simulink model "SecRwLtStCalib"  (R2024b)
settings: Solver=FixedStepDiscrete  StartTime=0.0  StopTime=10.0  FixedStep=0.01  RelTol=1e-3
model workspace (MAT data in the model file):
  KeSMSwAcsMd6SecRwLtStBkReclnUpwdDnwdPos1Max_Val = Simulink.Parameter
  KeSMSwAcsMd6SecRwLtStBkReclnUpwdDnwdPos1Max_Val.Value = 1960
  KeSMSwAcsMd6SecRwLtStBkReclnUpwdDnwdPos1Max_Val.Complexity = 'real'
  KeSMSwAcsMd6SecRwLtStBkReclnUpwdDnwdPos1Max_Val.Dimensions = [1 1]
  KeSMSwAcsMd6SecRwLtStBkReclnUpwdDnwdPos1Max_Val.DataType = 'uint16'
  KeSMSwAcsMd6SecRwLtStBkReclnUpwdDnwdPos1Min_Val = Simulink.Parameter
  KeSMSwAcsMd6SecRwLtStBkReclnUpwdDnwdPos1Min_Val.Value = 1960
  KeSMSwAcsMd6SecRwLtStBkReclnUpwdDnwdPos1Min_Val.Complexity = 'real'
  KeSMSwAcsMd6SecRwLtStBkReclnUpwdDnwdPos1Min_Val.Dimensions = [1 1]
  KeSMSwAcsMd6SecRwLtStBkReclnUpwdDnwdPos1Min_Val.DataType = 'uint16'
  KeSMSwAcsMd6SecRwLtStBkReclnUpwdDnwdPos1_Val = Simulink.Parameter
  KeSMSwAcsMd6SecRwLtStBkReclnUpwdDnwdPos1_Val.Value = 1960
  KeSMSwAcsMd6SecRwLtStBkReclnUpwdDnwdPos1_Val.Complexity = 'real'
  KeSMSwAcsMd6SecRwLtStBkReclnUpwdDnwdPos1_Val.Dimensions = [1 1]
  KeSMSwAcsMd6SecRwLtStBkReclnUpwdDnwdPos1_Val.DataType = 'uint16'
  KeSMSwAcsMd6SecRwLtStBkReclnUpwdDnwdPosMax_Val = Simulink.Parameter
  KeSMSwAcsMd6SecRwLtStBkReclnUpwdDnwdPosMax_Val.Value = 1960
  KeSMSwAcsMd6SecRwLtStBkReclnUpwdDnwdPosMax_Val.Complexity = 'real'
  KeSMSwAcsMd6SecRwLtStBkReclnUpwdDnwdPosMax_Val.Dimensions = [1 1]
  KeSMSwAcsMd6SecRwLtStBkReclnUpwdDnwdPosMax_Val.DataType = 'uint16'
  KeSMSwAcsMd6SecRwLtStBkReclnUpwdDnwdPosMin_Val = Simulink.Parameter
  KeSMSwAcsMd6SecRwLtStBkReclnUpwdDnwdPosMin_Val.Value = 1960
  KeSMSwAcsMd6SecRwLtStBkReclnUpwdDnwdPosMin_Val.Complexity = 'real'
  KeSMSwAcsMd6SecRwLtStBkReclnUpwdDnwdPosMin_Val.Dimensions = [1 1]
  KeSMSwAcsMd6SecRwLtStBkReclnUpwdDnwdPosMin_Val.DataType = 'uint16'
  KeSMSwAcsMd6SecRwLtStBkReclnUpwdDnwdPos_Val = Simulink.Parameter
  KeSMSwAcsMd6SecRwLtStBkReclnUpwdDnwdPos_Val.Value = 1960
  KeSMSwAcsMd6SecRwLtStBkReclnUpwdDnwdPos_Val.Complexity = 'real'
  KeSMSwAcsMd6SecRwLtStBkReclnUpwdDnwdPos_Val.Dimensions = [1 1]
  KeSMSwAcsMd6SecRwLtStBkReclnUpwdDnwdPos_Val.DataType = 'uint16'
undefined symbols (not defined in the file or in its folder): KeSMSw4SAcsMd21SecRwLtStBkReclnUpwdDnwdPos_Val, KeSMSw4SAcsMd21SecRwLtStBkReclnUpwdDnwdPosMax_Val, KeSMSw4SAcsMd21SecRwLtStBkReclnUpwdDnwdPosMin_Val, KeSMSw4SAcsMd21SecRwLtStFrwdBkwdPos_Val, KeSMSw4SAcsMd21SecRwLtStFrwdBkwdPosMax_Val, KeSMSw4SAcsMd21SecRwLtStFrwdBkwdPosMin_Val, KeSMSw4SAcsMd21SecRwLtStHdrstFrwdBkwdPos_Val, KeSMSw4SAcsMd21SecRwLtStHdrstFrwdBkwdPosMax_Val, KeSMSw4SAcsMd21SecRwLtStHdrstFrwdBkwdPosMin_Val, KeSMSw4SAcsMd21SecRwLtStHdrstUpwdDnwdPos_Val, KeSMSw4SAcsMd21SecRwLtStHdrstUpwdDnwdPosMax_Val, KeSMSw4SAcsMd21SecRwLtStHdrstUpwdDnwdPosMin_Val, KeSMSw4SAcsMd22SecRwLtStBkReclnUpwdDnwdPos1_Val, KeSMSw4SAcsMd22SecRwLtStBkReclnUpwdDnwdPos2_Val, KeSMSw4SAcsMd22SecRwLtStBkReclnUpwdDnwdPos2Max_Val, KeSMSw4SAcsMd22SecRwLtStBkReclnUpwdDnwdPos2Min_Val, KeSMSw4SAcsMd22SecRwLtStBkReclnUpwdDnwdPosMax_Val, KeSMSw4SAcsMd22SecRwLtStBkReclnUpwdDnwdPosMin_Val, KeSMSw4SAcsMd22SecRwLtStFrwdBkwdPos_Val, KeSMSw4SAcsMd22SecRwLtStFrwdBkwdPosMax_Val, KeSMSw4SAcsMd22SecRwLtStFrwdBkwdPosMin_Val, KeSMSw4SAcsMd22SecRwLtStFtrstUpwdDnwdPos_Val, KeSMSw4SAcsMd22SecRwLtStFtrstUpwdDnwdPosMax_Val, KeSMSw4SAcsMd22SecRwLtStFtrstUpwdDnwdPosMin_Val, KeSMSw4SAcsMd22SecRwLtStHdrstFrwdBkwdPos_Val, KeSMSw4SAcsMd22SecRwLtStHdrstFrwdBkwdPosMax_Val, KeSMSw4SAcsMd22SecRwLtStHdrstFrwdBkwdPosMin_Val, KeSMSw4SAcsMd22SecRwLtStHdrstUpwdDnwdPos_Val, KeSMSw4SAcsMd22SecRwLtStHdrstUpwdDnwdPosMax_Val, KeSMSw4SAcsMd22SecRwLtStHdrstUpwdDnwdPosMin_Val, KeSMSw4SAcsMd22SecRwLtStLegrstOtwdInwdPos_Val, KeSMSw4SAcsMd22SecRwLtStLegrstOtwdInwdPosMax_Val, KeSMSw4SAcsMd22SecRwLtStLegrstOtwdInwdPosMin_Val, KeSMSw4SAcsMd22SecRwLtStLegrstUpwdDnwdPos_Val, KeSMSw4SAcsMd22SecRwLtStLegrstUpwdDnwdPosMax_Val, KeSMSw4SAcsMd22SecRwLtStLegrstUpwdDnwdPosMin_Val, KeSMSw4SAcsMd25SecRwLtStBkReclnUpwdDnwdPos_Val, KeSMSw4SAcsMd25SecRwLtStBkReclnUpwdDnwdPosMax_Val, KeSMSw4SAcsMd25SecRwLtStBkReclnUpwdDnwdPosMin_Val, KeSMSw4SAcsMd25SecRwLtStFrwdBkwdPos_Val, KeSMSw4SAcsMd25SecRwLtStFrwdBkwdPosMax_Val, KeSMSw4SAcsMd25SecRwLtStFrwdBkwdPosMin_Val, KeSMSw4SAcsMd25SecRwLtStHdrstFrwdBkwdPos_Val, KeSMSw4SAcsMd25SecRwLtStHdrstFrwdBkwdPosMax_Val, KeSMSw4SAcsMd25SecRwLtStHdrstFrwdBkwdPosMin_Val, KeSMSw4SAcsMd25SecRwLtStHdrstUpwdDnwdPos_Val, KeSMSw4SAcsMd25SecRwLtStHdrstUpwdDnwdPosMax_Val, KeSMSw4SAcsMd25SecRwLtStHdrstUpwdDnwdPosMin_Val, KeSMSw4SAcsMd26SecRwLtStBkReclnUpwdDnwdPos_Val, KeSMSw4SAcsMd26SecRwLtStBkReclnUpwdDnwdPosMax_Val, KeSMSw4SAcsMd26SecRwLtStBkReclnUpwdDnwdPosMin_Val, KeSMSw4SAcsMd26SecRwLtStFrwdBkwdPos_Val, KeSMSw4SAcsMd26SecRwLtStFrwdBkwdPosMax_Val, KeSMSw4SAcsMd26SecRwLtStFrwdBkwdPosMin_Val, KeSMSw4SAcsMd26SecRwLtStFtrstUpwdDnwdPos_Val, KeSMSw4SAcsMd26SecRwLtStFtrstUpwdDnwdPosMax_Val, KeSMSw4SAcsMd26SecRwLtStFtrstUpwdDnwdPosMin_Val, KeSMSw4SAcsMd26SecRwLtStHdrstFrwdBkwdPos_Val, KeSMSw4SAcsMd26SecRwLtStHdrstFrwdBkwdPosMax_Val, KeSMSw4SAcsMd26SecRwLtStHdrstFrwdBkwdPosMin_Val ... (+496)
libraries: TrgtPosSelcLib x61, StIsPosChkLib x1, simulink x1
(part 1 of 8)
settings Model: ParameterArgumentNames=KeSMSwAcsMd6SecRwLtStBkReclnUpwdDnwdPos1Max_Val,KeSMSwAcsMd6SecRwLtStBkReclnUpwdDnwdPos1Min_Val,KeSMSwAcsMd6SecRwLtStBkReclnUpwdDnwdPos1_Val,KeSMSwAcsMd6SecRwLtStBkReclnUpwdDnwdPosMax_Val,KeSMSwAcsMd6SecRwLtStBkReclnUpwdDnwdPosMin_Val,KeSMSwAcsMd6SecRwLtStBkReclnUpwdDnwdPos_Val  Creator=sn2xws  LastModifiedBy=sn55gm
settings Model: ModifiedHistory=|
  | 2024.10.15 V3.0.0 新增Bitmask接口
  | 2024.10.29 V3.0.1 6s版本Md1 Md56靠背不应选择Cal1
  | 2024.12.12 V3.0.2 增加三排靠背折叠的判断余量
  | 25.7.1 V3.13.0 增加Md61 Md62
settings SolverCC: AlgebraicLoopSolver=TrustRegion
settings DataIOCC: SaveFormat=StructureWithTime  ReturnWorkspaceOutputs=off
settings OptimizationCC: DefaultParameterBehavior=Inlined  EnhancedBackFolding=on  PassReuseOutputArgsAs=Individual arguments  ZeroExternalMemoryAtStartup=off  ZeroInternalMemoryAtStartup=off  OptimizeBlockOrder=speed  DifferentSizesBufferReuse=on  OptimizationCustomize=off  EfficientTunableParamExpr=on
settings DebuggingCC: ParameterTunabilityLossMsg=error  UnconnectedInputMsg=warning  UnconnectedOutputMsg=warning  UnconnectedLineMsg=warning  ArithmeticOperatorsInVariantConditions=warning
settings ModelReferenceCC: EnableRefExpFcnMdlSchedulingChecks=on  ModelReferenceNumInstancesAllowed=Single
settings SFSimCC: MATLABDynamicMemAlloc=off  CustomCodeUndefinedFunction=UseInterfaceOnly
settings RTWCC: Description=AUTOSAR  SystemTargetFile=autosar.tlc  GenCodeOnly=on  TemplateMakefile=ert_default_tmf  GenerateReport=on  IncludeHyperlinkInReport=on  LaunchReport=on  DataTypeReplacement=CDataTypesFixedWidth  GenerateTraceInfo=on  GenerateTraceReport=on  GenerateTraceReportSl=on  GenerateTraceReportSf=on  GenerateTraceReportEml=on  GPUComputeCapability=3.5
settings CodeAppCC: ForceParamTrailComments=on  IgnoreCustomStorageClasses=off  OperatorAnnotations=on  SimulinkDataObjDesc=on  SFDataObjDesc=on  InsertBlockDesc=on
settings STFCustomTargetCC: TargetLangStandard=C99 (ISO)  MultiwordLength=256  ParMdlRefBuildCompliant=on  CompOptLevelCompliant=on  IncludeMdlTerminateFcn=off  CombineOutputUpdateFcns=on  SuppressErrorStatus=on  ERTCustomFileBanners=on  SupportNonFinite=off  SupportComplex=off  SupportContinuousTime=off  SupportNonInlinedSFcns=off  RemoveResetFunc=on  MATLABClassNameForMDSCustomization=Simulink.SoftwareTarget.ERTCustomization  AutosarCompliant=on  UseToolchainInfoCompliant=on  LookupTableObjectStructAxisOrder=2,1,3,4,...  LUTObjectStructOrderEvenSpacing=Size,Table,Breakpoints  SystemTargetFile=autosar.tlc
settings ERTTargetCC: TargetLangStandard=C99 (ISO)  ConcurrentExecutionCompliant=off  IncludeMdlTerminateFcn=off  SuppressErrorStatus=on  SupportNonFinite=off  SupportComplex=off  ModelStepFunctionPrototypeControlCompliant=off  CPPClassGenCompliant=off  AutosarCompliant=on  LookupTableObjectStructAxisOrder=2,1,3,4,...  LUTObjectStructOrderEvenSpacing=Size,Table,Breakpoints  ERTCustomFileTemplate=example_file_process.tlc  ERTFilePackagingFormat=Compact  BooleanTrueId=TRUE  BooleanFalseId=FALSE  DynamicArrayContainerType=coder::array

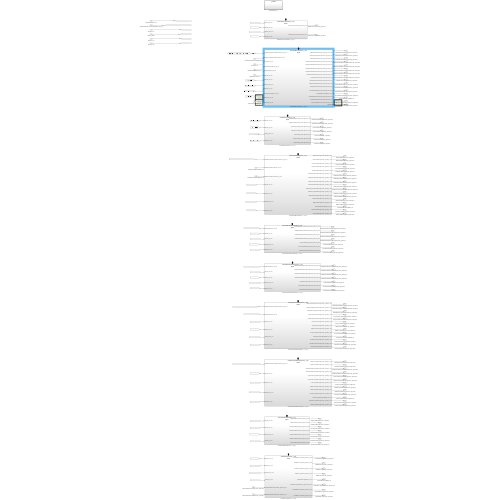
[thumbnail: Simulink's stored preview of the top-level diagram]
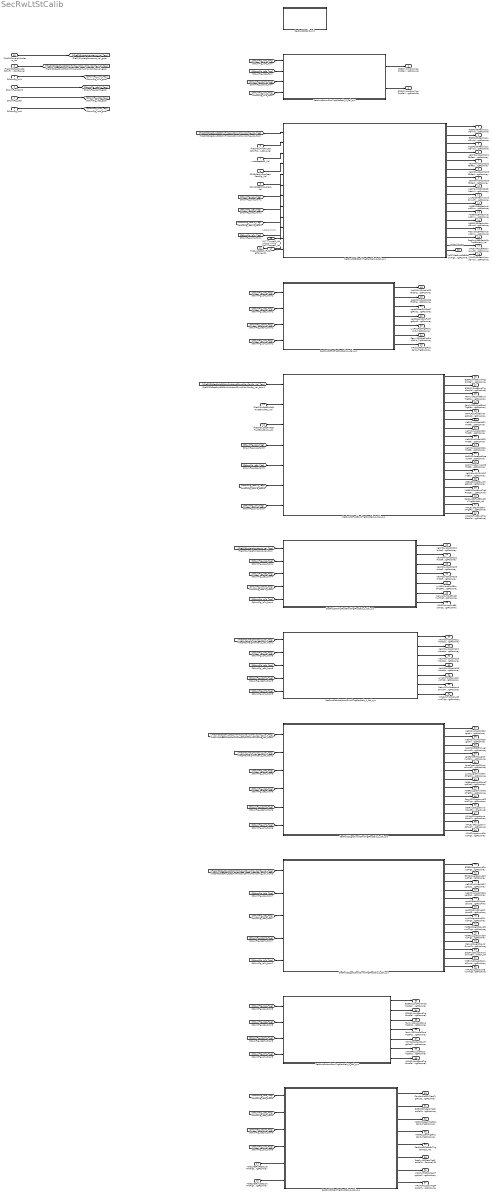
== system SecRwLtStCalib ==
  note: Added blocks
  note: Added blocks
  note: Added blocks
  StNumFlg_Is4s : Inport  OutDataTypeStr=boolean  PortDimensions=1
  StNumFlg_Is6s : Inport  Port=2  OutDataTypeStr=boolean  PortDimensions=1
  StNumFlg_Is6s7s : Inport  Port=3  OutDataTypeStr=boolean  PortDimensions=1
  StNumFlg_Is7s : Inport  Port=4  OutDataTypeStr=boolean  PortDimensions=1
  IfVeSMSbSecRwLtStCshnFrntUpwdDnwdMovConfig_Val : Inport  Port=5  OutDataTypeStr=boolean  PortDimensions=1
  IfVeSMSuThdRwLtStCshnFldUpwdDnwdPos_Val : Inport  Port=6  OutDataTypeStr=uint16  PortDimensions=1
  modestate32_Val : Inport  Port=7  OutDataTypeStr=uint32  PortDimensions=1
  R2LBkReclinFirstStepPassFlg_Val : Inport  Port=8  OutDataTypeStr=boolean  PortDimensions=1
  R2LMdSeatOccupied_Val : Inport  Port=9  OutDataTypeStr=boolean  PortDimensions=1
  ThdRwLtStCshnFldStgDone_Val : Inport  Port=10  OutDataTypeStr=boolean  PortDimensions=1
  IfVeSMSuSecRwRtStFrwdBkwdPos_Val : Inport  Port=11  OutDataTypeStr=uint16  PortDimensions=1
  IfVeSMSuSecRwRtStFrwdBkwdPosV_Val : Inport  Port=12  OutDataTypeStr=boolean  PortDimensions=1
  IfVeSMSuHeightIndexLt_Val : Inport  Description=|  Port=13  OutDataTypeStr=uint8  PortDimensions=1
      | 0：under 160
      | 1：160
      | 2：165
      | 3：170
      | 4：175
      | 5：180
      | 6：over 180
  Md61SecRwRtStCushFrntTrgtPosCalib_TrgtPosArray : Inport  Description=|  Port=14  OutDataTypeStr=uint16  PortDimensions=3
      | 0:Pos
      | 1:Max
      | 2:Min
  Md62SecRwLtStCushFrntTrgtPosCalib_TrgtPosArray : Inport  Description=|  Port=15  OutDataTypeStr=uint16  PortDimensions=3
      | 0:Pos
      | 1:Max
      | 2:Min
  Md27Target1_Val : Inport  Port=16  OutDataTypeStr=boolean  PortDimensions=1
  Md27Target2_Val : Inport  Port=17  OutDataTypeStr=boolean  PortDimensions=1
  SecRwLtStArmScrnTrgtPosSelc_1_Cal_sys : Subsystem
  SecRwLtStBkReclnTrgtPosSelc_1_Cal_sys : Subsystem
  SecRwLtStCalib_Init : Subsystem
  SecRwLtStFtrstTrgtPosSelc_1_Cal_sys : Subsystem
  SecRwLtStFwdBkwdTrgtPosSelc_1_Cal_sys : Subsystem
  SecRwLtStHdrstFwdBkwdTrgtPosSelc_1_Cal_sys : Subsystem
  SecRwLtStHdrstUpwdDnwdTrgtPosSelc_1_Cal_sys : Subsystem
  SecRwLtStLgrstInwdOtwdTrgtPosSelc_1_Cal_sys : Subsystem
  SecRwLtStLgrstUpwdDnwdTrgtPosSelc_1_Cal_sys : Subsystem
  SecRwLtStLtwdRtwdTrgtPosSelc_1_Cal_sys : Subsystem
  SecRwLtStZeroTrgtPosSelc_1_Cal_sys : Subsystem
  EZER2LArmScrnTrgtPosCalib_TrgtPosArray : Outport  Description=|  OutDataTypeStr=uint16  PortDimensions=3  VectorParamsAs1DForOutWhenUnconnected=off
      | 0:Pos
      | 1:Max
      | 2:Min
  EZQR2LArmScrnTrgtPosCalib_TrgtPosArray : Outport  Description=|  Port=2  OutDataTypeStr=uint16  PortDimensions=3  VectorParamsAs1DForOutWhenUnconnected=off
      | 0:Pos
      | 1:Max
      | 2:Min
  EZER2LBkReclnUpwdDnwdTrgtPosCalib_TrgtPosArray : Outport  Description=|  Port=3  OutDataTypeStr=uint16  PortDimensions=3  VectorParamsAs1DForOutWhenUnconnected=off
      | 0:Pos
      | 1:Max
      | 2:Min
  EZER2LBkReclnUpwdDnwdTrgtPosCalib1_TrgtPosArray : Outport  Description=|  Port=4  OutDataTypeStr=uint16  PortDimensions=3  VectorParamsAs1DForOutWhenUnconnected=off
      | 0:Pos
      | 1:Max
      | 2:Min
  EZQR2LBkReclnUpwdDnwdTrgtPosCalib_TrgtPosArray : Outport  Description=|  Port=5  OutDataTypeStr=uint16  PortDimensions=3  VectorParamsAs1DForOutWhenUnconnected=off
      | 0:Pos
      | 1:Max
      | 2:Min
  KeSMSw4SAcsMd21BkReclnUpwdDnwdTrgtPosCalib_TrgtPosArray : Outport  Description=|  Port=6  OutDataTypeStr=uint16  PortDimensions=3  VectorParamsAs1DForOutWhenUnconnected=off
      | 0:Pos
      | 1:Max
      | 2:Min
  KeSMSw4SAcsMd22BkReclnUpwdDnwdTrgtPosCalib_TrgtPosArray : Outport  Description=|  Port=7  OutDataTypeStr=uint16  PortDimensions=3  VectorParamsAs1DForOutWhenUnconnected=off
      | 0:Pos
      | 1:Max
      | 2:Min
  KeSMSw4SAcsMd25BkReclnUpwdDnwdTrgtPosCalib_TrgtPosArray : Outport  Description=|  Port=8  OutDataTypeStr=uint16  PortDimensions=3  VectorParamsAs1DForOutWhenUnconnected=off
      | 0:Pos
      | 1:Max
      | 2:Min
  KeSMSw4SAcsMd26BkReclnUpwdDnwdTrgtPosCalib_TrgtPosArray : Outport  Description=|  Port=9  OutDataTypeStr=uint16  PortDimensions=3  VectorParamsAs1DForOutWhenUnconnected=off
      | 0:Pos
      | 1:Max
      | 2:Min
  KeSMSwMd32R2LBkReclnUpwdDnwdTrgtPosCalib_TrgtPosArray : Outport  Description=|  Port=10  OutDataTypeStr=uint16  PortDimensions=3  VectorParamsAs1DForOutWhenUnconnected=off
      | 0:Pos
      | 1:Max
      | 2:Min
  LyLR2LBkReclnUpwdDnwdTrgtPosCalib_TrgtPosArray : Outport  Description=|  Port=11  OutDataTypeStr=uint16  PortDimensions=3  VectorParamsAs1DForOutWhenUnconnected=off
      | 0:Pos
      | 1:Max
      | 2:Min
  Md56R2LBkReclnUpwdDnwdTrgtPosCalib_TrgtPosArray : Outport  Description=|  Port=12  OutDataTypeStr=uint16  PortDimensions=3  VectorParamsAs1DForOutWhenUnconnected=off
      | 0:Pos
      | 1:Max
      | 2:Min
  Md56R2LBkReclnUpwdDnwdTrgtPosCalib1_TrgtPosArray : Outport  Description=|  Port=13  OutDataTypeStr=uint16  PortDimensions=3  VectorParamsAs1DForOutWhenUnconnected=off
      | 0:Pos
      | 1:Max
      | 2:Min
  Md8R2LBkReclnUpwdDnwdTrgtPosCalib_TrgtPosArray : Outport  Description=|  Port=14  OutDataTypeStr=uint16  PortDimensions=3  VectorParamsAs1DForOutWhenUnconnected=off
      | 0:Pos
      | 1:Max
      | 2:Min
  RecvLR2LBkReclnUpwdDnwdTrgtPosCalib_TrgtPosArray : Outport  Description=|  Port=15  OutDataTypeStr=uint16  PortDimensions=3  VectorParamsAs1DForOutWhenUnconnected=off
      | 0:Pos
      | 1:Max
      | 2:Min
  SecRwLtStBkReclnEnTrigBitMask_Val : Outport  Port=16  OutDataTypeStr=uint32  PortDimensions=1  VectorParamsAs1DForOutWhenUnconnected=off
  VIPLExitR2LBkReclnUpwdDnwdTrgtPosCalib_TrgtPosArray : Outport  Description=|  Port=17  OutDataTypeStr=uint16  PortDimensions=3  VectorParamsAs1DForOutWhenUnconnected=off
      | 0:Pos
      | 1:Max
      | 2:Min
  VIPLR2LBkReclnUpwdDnwdTrgtPosCalib_TrgtPosArray : Outport  Description=|  Port=18  OutDataTypeStr=uint16  PortDimensions=3  VectorParamsAs1DForOutWhenUnconnected=off
      | 0:Pos
      | 1:Max
      | 2:Min
  KeSMSw4SAcsMd22FtrstTrgtPosCalib_TrgtPosArray : Outport  Description=|  Port=19  OutDataTypeStr=uint16  PortDimensions=3  VectorParamsAs1DForOutWhenUnconnected=off
      | 0:Pos
      | 1:Max
      | 2:Min
  KeSMSw4SAcsMd26FtrstTrgtPosCalib_TrgtPosArray : Outport  Description=|  Port=20  OutDataTypeStr=uint16  PortDimensions=3  VectorParamsAs1DForOutWhenUnconnected=off
      | 0:Pos
      | 1:Max
      | 2:Min
  LgrstCloseLR2LFtrstTrgtPosCalib_TrgtPosArray : Outport  Description=|  Port=21  OutDataTypeStr=uint16  PortDimensions=3  VectorParamsAs1DForOutWhenUnconnected=off
      | 0:Pos
      | 1:Max
      | 2:Min
  LgrstOpenLR2LFtrstTrgtPosCalib_TrgtPosArray : Outport  Description=|  Port=22  OutDataTypeStr=uint16  PortDimensions=3  VectorParamsAs1DForOutWhenUnconnected=off
      | 0:Pos
      | 1:Max
      | 2:Min
  LyLR2LFtrstTrgtPosCalib_TrgtPosArray : Outport  Description=|  Port=23  OutDataTypeStr=uint16  PortDimensions=3  VectorParamsAs1DForOutWhenUnconnected=off
      | 0:Pos
      | 1:Max
      | 2:Min
  RecvLR2LFtrstTrgtPosCalib_TrgtPosArray : Outport  Description=|  Port=24  OutDataTypeStr=uint16  PortDimensions=3  VectorParamsAs1DForOutWhenUnconnected=off
      | 0:Pos
      | 1:Max
      | 2:Min
  VIPLR2LFtrstTrgtPosCalib_TrgtPosArray : Outport  Description=|  Port=25  OutDataTypeStr=uint16  PortDimensions=3  VectorParamsAs1DForOutWhenUnconnected=off
      | 0:Pos
      | 1:Max
      | 2:Min
  EZER2LFwdBkwdTrgtPosCalib_TrgtPosArray : Outport  Description=|  Port=26  OutDataTypeStr=uint16  PortDimensions=3  VectorParamsAs1DForOutWhenUnconnected=off
      | 0:Pos
      | 1:Max
      | 2:Min
  EZQR2LFwdBkwdTrgtPosCalib_TrgtPosArray : Outport  Description=|  Port=27  OutDataTypeStr=uint16  PortDimensions=3  VectorParamsAs1DForOutWhenUnconnected=off
      | 0:Pos
      | 1:Max
      | 2:Min
  FamlyLR2LFwdBkwdTrgtPosCalib_TrgtPosArray : Outport  Description=|  Port=28  OutDataTypeStr=uint16  PortDimensions=3  VectorParamsAs1DForOutWhenUnconnected=off
      | 0:Pos
      | 1:Max
      | 2:Min
  FamlyRR2LFwdBkwdTrgtPosCalib_TrgtPosArray : Outport  Description=|  Port=29  OutDataTypeStr=uint16  PortDimensions=3  VectorParamsAs1DForOutWhenUnconnected=off
      | 0:Pos
      | 1:Max
      | 2:Min
  INTMLR2LFwdBkwdTrgtPosCalib_TrgtPosArray : Outport  Description=|  Port=30  OutDataTypeStr=uint16  PortDimensions=3  VectorParamsAs1DForOutWhenUnconnected=off
      | 0:Pos
      | 1:Max
      | 2:Min
  KeSMSw4SAcsMd21FwdBkwdTrgtPosCalib_TrgtPosArray : Outport  Description=|  Port=31  OutDataTypeStr=uint16  PortDimensions=3  VectorParamsAs1DForOutWhenUnconnected=off
      | 0:Pos
      | 1:Max
      | 2:Min
  KeSMSw4SAcsMd22FwdBkwdTrgtPosCalib_TrgtPosArray : Outport  Description=|  Port=32  OutDataTypeStr=uint16  PortDimensions=3  VectorParamsAs1DForOutWhenUnconnected=off
      | 0:Pos
      | 1:Max
      | 2:Min
  KeSMSw4SAcsMd25FwdBkwdTrgtPosCalib_TrgtPosArray : Outport  Description=|  Port=33  OutDataTypeStr=uint16  PortDimensions=3  VectorParamsAs1DForOutWhenUnconnected=off
      | 0:Pos
      | 1:Max
      | 2:Min
  KeSMSw4SAcsMd26FwdBkwdTrgtPosCalib_TrgtPosArray : Outport  Description=|  Port=34  OutDataTypeStr=uint16  PortDimensions=3  VectorParamsAs1DForOutWhenUnconnected=off
      | 0:Pos
      | 1:Max
      | 2:Min
  KeSMSw4sLegrstOpenLMdFwdBkwdTrgtPosCalib_TrgtPosArray : Outport  Description=|  Port=35  OutDataTypeStr=uint16  PortDimensions=3  VectorParamsAs1DForOutWhenUnconnected=off
      | 0:Pos
      | 1:Max
      | 2:Min
  KeSMSw4SLyingLMDFwdBkwdTrgtPosCalib_TrgtPosArray : Outport  Description=|  Port=36  OutDataTypeStr=uint16  PortDimensions=3  VectorParamsAs1DForOutWhenUnconnected=off
      | 0:Pos
      | 1:Max
      | 2:Min
  KeSMSw4SVIPLMDFwdBkwdTrgtPosCalib_TrgtPosArray : Outport  Description=|  Port=37  OutDataTypeStr=uint16  PortDimensions=3  VectorParamsAs1DForOutWhenUnconnected=off
      | 0:Pos
      | 1:Max
      | 2:Min
  Md56R2LFwdBkwdTrgtPosCalib_TrgtPosArray : Outport  Description=|  Port=38  OutDataTypeStr=uint16  PortDimensions=3  VectorParamsAs1DForOutWhenUnconnected=off
      | 0:Pos
      | 1:Max
      | 2:Min
  Md8R2LFwdBkwdTrgtPosCalib_TrgtPosArray : Outport  Description=|  Port=39  OutDataTypeStr=uint16  PortDimensions=3  VectorParamsAs1DForOutWhenUnconnected=off
      | 0:Pos
      | 1:Max
      | 2:Min
  SecRwLtStFwdBkwdEnTrigBitMask_Val : Outport  Port=40  OutDataTypeStr=uint32  PortDimensions=1  VectorParamsAs1DForOutWhenUnconnected=off
  VIPLExitR2LFwdBkwdTrgtPosCalib_TrgtPosArray : Outport  Description=|  Port=41  OutDataTypeStr=uint16  PortDimensions=3  VectorParamsAs1DForOutWhenUnconnected=off
      | 0:Pos
      | 1:Max
      | 2:Min
  VIPLR2LFwdBkwdTrgtPosCalib_TrgtPosArray : Outport  Description=|  Port=42  OutDataTypeStr=uint16  PortDimensions=3  VectorParamsAs1DForOutWhenUnconnected=off
      | 0:Pos
      | 1:Max
      | 2:Min
  KeSMSw4SAcsMd21HdrstFwdBkwdTrgtPosCalib_TrgtPosArray : Outport  Description=|  Port=43  OutDataTypeStr=uint16  PortDimensions=3  VectorParamsAs1DForOutWhenUnconnected=off
      | 0:Pos
      | 1:Max
      | 2:Min
  KeSMSw4SAcsMd22HdrstFwdBkwdTrgtPosCalib_TrgtPosArray : Outport  Description=|  Port=44  OutDataTypeStr=uint16  PortDimensions=3  VectorParamsAs1DForOutWhenUnconnected=off
      | 0:Pos
      | 1:Max
      | 2:Min
  KeSMSw4SAcsMd25HdrstFwdBkwdTrgtPosCalib_TrgtPosArray : Outport  Description=|  Port=45  OutDataTypeStr=uint16  PortDimensions=3  VectorParamsAs1DForOutWhenUnconnected=off
      | 0:Pos
      | 1:Max
      | 2:Min
  KeSMSw4SAcsMd26HdrstFwdBkwdTrgtPosCalib_TrgtPosArray : Outport  Description=|  Port=46  OutDataTypeStr=uint16  PortDimensions=3  VectorParamsAs1DForOutWhenUnconnected=off
      | 0:Pos
      | 1:Max
      | 2:Min
  LyLR2LHdrstFwdBkwdTrgtPosCalib_TrgtPosArray : Outport  Description=|  Port=47  OutDataTypeStr=uint16  PortDimensions=3  VectorParamsAs1DForOutWhenUnconnected=off
      | 0:Pos
      | 1:Max
      | 2:Min
  RecvLR2LHdrstFwdBkwdTrgtPosCalib_TrgtPosArray : Outport  Description=|  Port=48  OutDataTypeStr=uint16  PortDimensions=3  VectorParamsAs1DForOutWhenUnconnected=off
      | 0:Pos
      | 1:Max
      | 2:Min
  VIPLR2LHdrstFwdBkwdTrgtPosCalib_TrgtPosArray : Outport  Description=|  Port=49  OutDataTypeStr=uint16  PortDimensions=3  VectorParamsAs1DForOutWhenUnconnected=off
      | 0:Pos
      | 1:Max
      | 2:Min
  KeSMSw4SAcsMd21HdrstUpwdDnwdTrgtPosCalib_TrgtPosArray : Outport  Description=|  Port=50  OutDataTypeStr=uint16  PortDimensions=3  VectorParamsAs1DForOutWhenUnconnected=off
      | 0:Pos
      | 1:Max
      | 2:Min
  KeSMSw4SAcsMd22HdrstUpwdDnwdTrgtPosCalib_TrgtPosArray : Outport  Description=|  Port=51  OutDataTypeStr=uint16  PortDimensions=3  VectorParamsAs1DForOutWhenUnconnected=off
      | 0:Pos
      | 1:Max
      | 2:Min
  KeSMSw4SAcsMd25HdrstUpwdDnwdTrgtPosCalib_TrgtPosArray : Outport  Description=|  Port=52  OutDataTypeStr=uint16  PortDimensions=3  VectorParamsAs1DForOutWhenUnconnected=off
      | 0:Pos
      | 1:Max
      | 2:Min
  KeSMSw4SAcsMd26HdrstUpwdDnwdTrgtPosCalib_TrgtPosArray : Outport  Description=|  Port=53  OutDataTypeStr=uint16  PortDimensions=3  VectorParamsAs1DForOutWhenUnconnected=off
      | 0:Pos
      | 1:Max
      | 2:Min
  LyLR2LHdrstUpwdDnwdTrgtPosCalib_TrgtPosArray : Outport  Description=|  Port=54  OutDataTypeStr=uint16  PortDimensions=3  VectorParamsAs1DForOutWhenUnconnected=off
      | 0:Pos
      | 1:Max
      | 2:Min
  RecvLR2LHdrstUpwdDnwdTrgtPosCalib_TrgtPosArray : Outport  Description=|  Port=55  OutDataTypeStr=uint16  PortDimensions=3  VectorParamsAs1DForOutWhenUnconnected=off
      | 0:Pos
      | 1:Max
      | 2:Min
  VIPLR2LHdrstUpwdDnwdTrgtPosCalib_TrgtPosArray : Outport  Description=|  Port=56  OutDataTypeStr=uint16  PortDimensions=3  VectorParamsAs1DForOutWhenUnconnected=off
      | 0:Pos
      | 1:Max
      | 2:Min
  KeSMSw4SAcsMd22LgrstInwdOtwdTrgtPosCalib_TrgtPosArray : Outport  Description=|  Port=57  OutDataTypeStr=uint16  PortDimensions=3  VectorParamsAs1DForOutWhenUnconnected=off
      | 0:Pos
      | 1:Max
      | 2:Min
  KeSMSw4SAcsMd26LgrstInwdOtwdTrgtPosCalib_TrgtPosArray : Outport  Description=|  Port=58  OutDataTypeStr=uint16  PortDimensions=3  VectorParamsAs1DForOutWhenUnconnected=off
      | 0:Pos
      | 1:Max
      | 2:Min
  KeSMSwEZEEntryLgrstInwdOtwdTrgtPosCalib_TrgtPosArray : Outport  Description=|  Port=59  OutDataTypeStr=uint16  PortDimensions=3  VectorParamsAs1DForOutWhenUnconnected=off
      | 0:Pos
      | 1:Max
      | 2:Min
  LgrstCloseLR2LLgrstInwdOtwdTrgtPosCalib_TrgtPosArray : Outport  Description=|  Port=60  OutDataTypeStr=uint16  PortDimensions=3  VectorParamsAs1DForOutWhenUnconnected=off
      | 0:Pos
      | 1:Max
      | 2:Min
  LgrstOpen4sLR2LLgrstInwdOtwdTrgtPosCalib_TrgtPosArray : Outport  Description=|  Port=61  OutDataTypeStr=uint16  PortDimensions=3  VectorParamsAs1DForOutWhenUnconnected=off
      | 0:Pos
      | 1:Max
      | 2:Min
  LyLR2LLgrstInwdOtwdTrgtPosCalib_TrgtPosArray : Outport  Description=|  Port=62  OutDataTypeStr=uint16  PortDimensions=3  VectorParamsAs1DForOutWhenUnconnected=off
      | 0:Pos
      | 1:Max
      | 2:Min
  Md56LgrstInwdOtwdTrgtPosCalib_TrgtPosArray : Outport  Description=|  Port=63  OutDataTypeStr=uint16  PortDimensions=3  VectorParamsAs1DForOutWhenUnconnected=off
      | 0:Pos
      | 1:Max
      | 2:Min
  Md8R2LLgrstInwdOtwdTrgtPosCalib_TrgtPosArray : Outport  Description=|  Port=64  OutDataTypeStr=uint16  PortDimensions=3  VectorParamsAs1DForOutWhenUnconnected=off
      | 0:Pos
      | 1:Max
      | 2:Min
  RecvLR2LLgrstInwdOtwdTrgtPosCalib_TrgtPosArray : Outport  Description=|  Port=65  OutDataTypeStr=uint16  PortDimensions=3  VectorParamsAs1DForOutWhenUnconnected=off
      | 0:Pos
      | 1:Max
      | 2:Min
  SecRwLtStLgrstInwdOtwdEnTrigBitMask_Val : Outport  Port=66  OutDataTypeStr=uint32  PortDimensions=1  VectorParamsAs1DForOutWhenUnconnected=off
  VIP4sLR2LLgrstInwdOtwdTrgtPosCalib_TrgtPosArray : Outport  Description=|  Port=67  OutDataTypeStr=uint16  PortDimensions=3  VectorParamsAs1DForOutWhenUnconnected=off
      | 0:Pos
      | 1:Max
      | 2:Min
  VIPLExitR2LLgrstInwdOtwdTrgtPosCalib_TrgtPosArray : Outport  Description=|  Port=68  OutDataTypeStr=uint16  PortDimensions=3  VectorParamsAs1DForOutWhenUnconnected=off
      | 0:Pos
      | 1:Max
      | 2:Min
  VIPLR2LLgrstInwdOtwdTrgtPosCalib_TrgtPosArray : Outport  Description=|  Port=69  OutDataTypeStr=uint16  PortDimensions=3  VectorParamsAs1DForOutWhenUnconnected=off
      | 0:Pos
      | 1:Max
      | 2:Min
  EZER2LLgrstUpwdDnwdTrgtPosCalib_TrgtPosArray : Outport  Description=|  Port=70  OutDataTypeStr=uint16  PortDimensions=3  VectorParamsAs1DForOutWhenUnconnected=off
      | 0:Pos
      | 1:Max
      | 2:Min
  EZQR2LLgrstUpwdDnwdTrgtPosCalib_TrgtPosArray : Outport  Description=|  Port=71  OutDataTypeStr=uint16  PortDimensions=3  VectorParamsAs1DForOutWhenUnconnected=off
      | 0:Pos
      | 1:Max
      | 2:Min
  KeSMSw4SAcsMd22LgrstUpwdDnwdTrgtPosCalib_TrgtPosArray : Outport  Description=|  Port=72  OutDataTypeStr=uint16  PortDimensions=3  VectorParamsAs1DForOutWhenUnconnected=off
      | 0:Pos
      | 1:Max
      | 2:Min
  KeSMSw4SAcsMd26LgrstUpwdDnwdTrgtPosCalib_TrgtPosArray : Outport  Description=|  Port=73  OutDataTypeStr=uint16  PortDimensions=3  VectorParamsAs1DForOutWhenUnconnected=off
      | 0:Pos
      | 1:Max
      | 2:Min
  LgrstCloseLR2LLgrstUpwdDnwdTrgtPosCalib_TrgtPosArray : Outport  Description=|  Port=74  OutDataTypeStr=uint16  PortDimensions=3  VectorParamsAs1DForOutWhenUnconnected=off
      | 0:Pos
      | 1:Max
      | 2:Min
  LgrstOpenLR2LLgrstUpwdDnwdTrgtPosCalib_TrgtPosArray : Outport  Description=|  Port=75  OutDataTypeStr=uint16  PortDimensions=3  VectorParamsAs1DForOutWhenUnconnected=off
      | 0:Pos
      | 1:Max
      | 2:Min
  LyLR2LLgrstUpwdDnwdTrgtPosCalib_TrgtPosArray : Outport  Description=|  Port=76  OutDataTypeStr=uint16  PortDimensions=3  VectorParamsAs1DForOutWhenUnconnected=off
      | 0:Pos
      | 1:Max
      | 2:Min
  Md56R2LLgrstUpwdDnwdTrgtPosCalib_TrgtPosArray : Outport  Description=|  Port=77  OutDataTypeStr=uint16  PortDimensions=3  VectorParamsAs1DForOutWhenUnconnected=off
      | 0:Pos
      | 1:Max
      | 2:Min
  Md8R2LLgrstUpwdDnwdTrgtPosCalib_TrgtPosArray : Outport  Description=|  Port=78  OutDataTypeStr=uint16  PortDimensions=3  VectorParamsAs1DForOutWhenUnconnected=off
      | 0:Pos
      | 1:Max
      | 2:Min
  RecvLR2LLgrstUpwdDnwdTrgtPosCalib_TrgtPosArray : Outport  Description=|  Port=79  OutDataTypeStr=uint16  PortDimensions=3  VectorParamsAs1DForOutWhenUnconnected=off
      | 0:Pos
      | 1:Max
      | 2:Min
  SecRwLtStLgrstUpwdDnwdEnTrigBitMask_Val : Outport  Port=80  OutDataTypeStr=uint32  PortDimensions=1  VectorParamsAs1DForOutWhenUnconnected=off
  VIPExitLR2LLgrstUpwdDnwdTrgtPosCalib_TrgtPosArray : Outport  Description=|  Port=81  OutDataTypeStr=uint16  PortDimensions=3  VectorParamsAs1DForOutWhenUnconnected=off
      | 0:Pos
      | 1:Max
      | 2:Min
  VIPLR2LLgrstUpwdDnwdTrgtPosCalib_TrgtPosArray : Outport  Description=|  Port=82  OutDataTypeStr=uint16  PortDimensions=3  VectorParamsAs1DForOutWhenUnconnected=off
      | 0:Pos
      | 1:Max
      | 2:Min
  EZER2LLtwdRtwdTrgtPosCalib_TrgtPosArray : Outport  Description=|  Port=83  OutDataTypeStr=uint16  PortDimensions=3  VectorParamsAs1DForOutWhenUnconnected=off
      | 0:Pos
      | 1:Max
      | 2:Min
  EZQR2LLtwdRtwdTrgtPosCalib_TrgtPosArray : Outport  Description=|  Port=84  OutDataTypeStr=uint16  PortDimensions=3  VectorParamsAs1DForOutWhenUnconnected=off
      | 0:Pos
      | 1:Max
      | 2:Min
  FamlyLR2LLtwdRtwdTrgtPosCalib_TrgtPosArray : Outport  Description=|  Port=85  OutDataTypeStr=uint16  PortDimensions=3  VectorParamsAs1DForOutWhenUnconnected=off
      | 0:Pos
      | 1:Max
      | 2:Min
  FamlyRR2LLtwdRtwdTrgtPosCalib_TrgtPosArray : Outport  Description=|  Port=86  OutDataTypeStr=uint16  PortDimensions=3  VectorParamsAs1DForOutWhenUnconnected=off
      | 0:Pos
      | 1:Max
      | 2:Min
  INTMLR2LLtwdRtwdTrgtPosCalib_TrgtPosArray : Outport  Description=|  Port=87  OutDataTypeStr=uint16  PortDimensions=3  VectorParamsAs1DForOutWhenUnconnected=off
      | 0:Pos
      | 1:Max
      | 2:Min
  INTMRR2LLtwdRtwdTrgtPosCalib_TrgtPosArray : Outport  Description=|  Port=88  OutDataTypeStr=uint16  PortDimensions=3  VectorParamsAs1DForOutWhenUnconnected=off
      | 0:Pos
      | 1:Max
      | 2:Min
  VIPLR2LLtwdRtwdTrgtPosCalib_TrgtPosArray : Outport  Description=|  Port=89  OutDataTypeStr=uint16  PortDimensions=3  VectorParamsAs1DForOutWhenUnconnected=off
      | 0:Pos
      | 1:Max
      | 2:Min
  ComfortMdR2LZeroTrgtPosCalib_TrgtPosArray : Outport  Description=|  Port=90  OutDataTypeStr=uint16  PortDimensions=3  VectorParamsAs1DForOutWhenUnconnected=off
      | 0:Pos
      | 1:Max
      | 2:Min
  EZEMdR2LZeroTrgtPosCalib_TrgtPosArray : Outport  Description=|  Port=91  OutDataTypeStr=uint16  PortDimensions=3  VectorParamsAs1DForOutWhenUnconnected=off
      | 0:Pos
      | 1:Max
      | 2:Min
  Md56R2LZeroTrgtPosCalib_TrgtPosArray : Outport  Description=|  Port=92  OutDataTypeStr=uint16  PortDimensions=3  VectorParamsAs1DForOutWhenUnconnected=off
      | 0:Pos
      | 1:Max
      | 2:Min
  Md8R2LZeroTrgtPosCalib_TrgtPosArray : Outport  Description=|  Port=93  OutDataTypeStr=uint16  PortDimensions=3  VectorParamsAs1DForOutWhenUnconnected=off
      | 0:Pos
      | 1:Max
      | 2:Min
  SecRwLtStZeroEnTrigBitMask_Val : Outport  Port=94  OutDataTypeStr=uint32  PortDimensions=1  VectorParamsAs1DForOutWhenUnconnected=off
  SecRwLtStZeroTrgtPosCalibArray32_TrgtPosArray32 : Outport  Description=|  Port=95  OutDataTypeStr=uint16  PortDimensions=96  VectorParamsAs1DForOutWhenUnconnected=off
      | 0:Pos
      | 1:Max
      | 2:Min
  VIPLExitMdR2LZeroTrgtPosCalib_TrgtPosArray : Outport  Description=|  Port=96  OutDataTypeStr=uint16  PortDimensions=3  VectorParamsAs1DForOutWhenUnconnected=off
      | 0:Pos
      | 1:Max
      | 2:Min
  VIPLMdR2LZeroTrgtPosCalib_TrgtPosArray : Outport  Description=|  Port=97  OutDataTypeStr=uint16  PortDimensions=3  VectorParamsAs1DForOutWhenUnconnected=off
      | 0:Pos
      | 1:Max
      | 2:Min
  Md27SecRwLtStBkReclnTrgtPosCalib_TrgtPosArray : Outport  Description=|  Port=98  OutDataTypeStr=uint16  PortDimensions=3  VectorParamsAs1DForOutWhenUnconnected=off
      | 0:Pos
      | 1:Max
      | 2:Min
  wires:
  SecRwLtStArmScrnTrgtPosSelc_1_Cal_sys/1(EZER2LArmScrnTrgtPosCalib_TrgtPosArray_write) -> EZER2LArmScrnTrgtPosCalib_TrgtPosArray/1
  SecRwLtStArmScrnTrgtPosSelc_1_Cal_sys/2(EZQR2LArmScrnTrgtPosCalib_TrgtPosArray_write) -> EZQR2LArmScrnTrgtPosCalib_TrgtPosArray/1
  IfVeSMSuThdRwLtStCshnFldUpwdDnwdPos_Val/1 -> SecRwLtStBkReclnTrgtPosSelc_1_Cal_sys/2(IfVeSMSuThdRwLtStCshnFldUpwdDnwdPos_Val_read)
  modestate32_Val/1 -> SecRwLtStBkReclnTrgtPosSelc_1_Cal_sys/3(modestate32_Val_read)
  R2LBkReclinFirstStepPassFlg_Val/1 -> SecRwLtStBkReclnTrgtPosSelc_1_Cal_sys/4(R2LBkReclinFirstStepPassFlg_Val_read)
  R2LMdSeatOccupied_Val/1 -> SecRwLtStBkReclnTrgtPosSelc_1_Cal_sys/5(R2LMdSeatOccupied_Val_read)
  ThdRwLtStCshnFldStgDone_Val/1 -> SecRwLtStBkReclnTrgtPosSelc_1_Cal_sys/10(ThdRwLtStCshnFldStgDone_Val_read)
  SecRwLtStBkReclnTrgtPosSelc_1_Cal_sys/1(EZER2LBkReclnUpwdDnwdTrgtPosCalib_TrgtPosArray_write) -> EZER2LBkReclnUpwdDnwdTrgtPosCalib_TrgtPosArray/1
  SecRwLtStBkReclnTrgtPosSelc_1_Cal_sys/2(EZER2LBkReclnUpwdDnwdTrgtPosCalib1_TrgtPosArray_write) -> EZER2LBkReclnUpwdDnwdTrgtPosCalib1_TrgtPosArray/1
  SecRwLtStBkReclnTrgtPosSelc_1_Cal_sys/3(EZQR2LBkReclnUpwdDnwdTrgtPosCalib_TrgtPosArray_write) -> EZQR2LBkReclnUpwdDnwdTrgtPosCalib_TrgtPosArray/1
  SecRwLtStBkReclnTrgtPosSelc_1_Cal_sys/4(KeSMSw4SAcsMd21BkReclnUpwdDnwdTrgtPosCalib_TrgtPosArray_write) -> KeSMSw4SAcsMd21BkReclnUpwdDnwdTrgtPosCalib_TrgtPosArray/1
  SecRwLtStBkReclnTrgtPosSelc_1_Cal_sys/5(KeSMSw4SAcsMd22BkReclnUpwdDnwdTrgtPosCalib_TrgtPosArray_write) -> KeSMSw4SAcsMd22BkReclnUpwdDnwdTrgtPosCalib_TrgtPosArray/1
  SecRwLtStBkReclnTrgtPosSelc_1_Cal_sys/6(KeSMSw4SAcsMd25BkReclnUpwdDnwdTrgtPosCalib_TrgtPosArray_write) -> KeSMSw4SAcsMd25BkReclnUpwdDnwdTrgtPosCalib_TrgtPosArray/1
  SecRwLtStBkReclnTrgtPosSelc_1_Cal_sys/7(KeSMSw4SAcsMd26BkReclnUpwdDnwdTrgtPosCalib_TrgtPosArray_write) -> KeSMSw4SAcsMd26BkReclnUpwdDnwdTrgtPosCalib_TrgtPosArray/1
  SecRwLtStBkReclnTrgtPosSelc_1_Cal_sys/8(KeSMSwMd32R2LBkReclnUpwdDnwdTrgtPosCalib_TrgtPosArray_write) -> KeSMSwMd32R2LBkReclnUpwdDnwdTrgtPosCalib_TrgtPosArray/1
  SecRwLtStBkReclnTrgtPosSelc_1_Cal_sys/9(LyLR2LBkReclnUpwdDnwdTrgtPosCalib_TrgtPosArray_write) -> LyLR2LBkReclnUpwdDnwdTrgtPosCalib_TrgtPosArray/1
  SecRwLtStBkReclnTrgtPosSelc_1_Cal_sys/10(Md56R2LBkReclnUpwdDnwdTrgtPosCalib_TrgtPosArray_write) -> Md56R2LBkReclnUpwdDnwdTrgtPosCalib_TrgtPosArray/1
  SecRwLtStBkReclnTrgtPosSelc_1_Cal_sys/11(Md56R2LBkReclnUpwdDnwdTrgtPosCalib1_TrgtPosArray_write) -> Md56R2LBkReclnUpwdDnwdTrgtPosCalib1_TrgtPosArray/1
  SecRwLtStBkReclnTrgtPosSelc_1_Cal_sys/12(Md8R2LBkReclnUpwdDnwdTrgtPosCalib_TrgtPosArray_write) -> Md8R2LBkReclnUpwdDnwdTrgtPosCalib_TrgtPosArray/1
  SecRwLtStBkReclnTrgtPosSelc_1_Cal_sys/13(RecvLR2LBkReclnUpwdDnwdTrgtPosCalib_TrgtPosArray_write) -> RecvLR2LBkReclnUpwdDnwdTrgtPosCalib_TrgtPosArray/1
  SecRwLtStBkReclnTrgtPosSelc_1_Cal_sys/14(SecRwLtStBkReclnEnTrigBitMask_Val_write) -> SecRwLtStBkReclnEnTrigBitMask_Val/1
  SecRwLtStBkReclnTrgtPosSelc_1_Cal_sys/15(VIPLExitR2LBkReclnUpwdDnwdTrgtPosCalib_TrgtPosArray_write) -> VIPLExitR2LBkReclnUpwdDnwdTrgtPosCalib_TrgtPosArray/1
  SecRwLtStBkReclnTrgtPosSelc_1_Cal_sys/16(VIPLR2LBkReclnUpwdDnwdTrgtPosCalib_TrgtPosArray_write) -> VIPLR2LBkReclnUpwdDnwdTrgtPosCalib_TrgtPosArray/1
  SecRwLtStFtrstTrgtPosSelc_1_Cal_sys/1(KeSMSw4SAcsMd22FtrstTrgtPosCalib_TrgtPosArray_write) -> KeSMSw4SAcsMd22FtrstTrgtPosCalib_TrgtPosArray/1
  SecRwLtStFtrstTrgtPosSelc_1_Cal_sys/2(KeSMSw4SAcsMd26FtrstTrgtPosCalib_TrgtPosArray_write) -> KeSMSw4SAcsMd26FtrstTrgtPosCalib_TrgtPosArray/1
  SecRwLtStFtrstTrgtPosSelc_1_Cal_sys/3(LgrstCloseLR2LFtrstTrgtPosCalib_TrgtPosArray_write) -> LgrstCloseLR2LFtrstTrgtPosCalib_TrgtPosArray/1
  SecRwLtStFtrstTrgtPosSelc_1_Cal_sys/4(LgrstOpenLR2LFtrstTrgtPosCalib_TrgtPosArray_write) -> LgrstOpenLR2LFtrstTrgtPosCalib_TrgtPosArray/1
  SecRwLtStFtrstTrgtPosSelc_1_Cal_sys/5(LyLR2LFtrstTrgtPosCalib_TrgtPosArray_write) -> LyLR2LFtrstTrgtPosCalib_TrgtPosArray/1
  SecRwLtStFtrstTrgtPosSelc_1_Cal_sys/6(RecvLR2LFtrstTrgtPosCalib_TrgtPosArray_write) -> RecvLR2LFtrstTrgtPosCalib_TrgtPosArray/1
  SecRwLtStFtrstTrgtPosSelc_1_Cal_sys/7(VIPLR2LFtrstTrgtPosCalib_TrgtPosArray_write) -> VIPLR2LFtrstTrgtPosCalib_TrgtPosArray/1
  IfVeSMSuSecRwRtStFrwdBkwdPos_Val/1 -> SecRwLtStFwdBkwdTrgtPosSelc_1_Cal_sys/2(IfVeSMSuSecRwRtStFrwdBkwdPos_Val_read)
  IfVeSMSuSecRwRtStFrwdBkwdPosV_Val/1 -> SecRwLtStFwdBkwdTrgtPosSelc_1_Cal_sys/3(IfVeSMSuSecRwRtStFrwdBkwdPosV_Val_read)
  SecRwLtStFwdBkwdTrgtPosSelc_1_Cal_sys/1(EZER2LFwdBkwdTrgtPosCalib_TrgtPosArray_write) -> EZER2LFwdBkwdTrgtPosCalib_TrgtPosArray/1
  SecRwLtStFwdBkwdTrgtPosSelc_1_Cal_sys/2(EZQR2LFwdBkwdTrgtPosCalib_TrgtPosArray_write) -> EZQR2LFwdBkwdTrgtPosCalib_TrgtPosArray/1
  SecRwLtStFwdBkwdTrgtPosSelc_1_Cal_sys/3(FamlyLR2LFwdBkwdTrgtPosCalib_TrgtPosArray_write) -> FamlyLR2LFwdBkwdTrgtPosCalib_TrgtPosArray/1
  SecRwLtStFwdBkwdTrgtPosSelc_1_Cal_sys/4(FamlyRR2LFwdBkwdTrgtPosCalib_TrgtPosArray_write) -> FamlyRR2LFwdBkwdTrgtPosCalib_TrgtPosArray/1
  SecRwLtStFwdBkwdTrgtPosSelc_1_Cal_sys/5(INTMLR2LFwdBkwdTrgtPosCalib_TrgtPosArray_write) -> INTMLR2LFwdBkwdTrgtPosCalib_TrgtPosArray/1
  SecRwLtStFwdBkwdTrgtPosSelc_1_Cal_sys/6(KeSMSw4SAcsMd21FwdBkwdTrgtPosCalib_TrgtPosArray_write) -> KeSMSw4SAcsMd21FwdBkwdTrgtPosCalib_TrgtPosArray/1
  SecRwLtStFwdBkwdTrgtPosSelc_1_Cal_sys/7(KeSMSw4SAcsMd22FwdBkwdTrgtPosCalib_TrgtPosArray_write) -> KeSMSw4SAcsMd22FwdBkwdTrgtPosCalib_TrgtPosArray/1
  SecRwLtStFwdBkwdTrgtPosSelc_1_Cal_sys/8(KeSMSw4SAcsMd25FwdBkwdTrgtPosCalib_TrgtPosArray_write) -> KeSMSw4SAcsMd25FwdBkwdTrgtPosCalib_TrgtPosArray/1
  SecRwLtStFwdBkwdTrgtPosSelc_1_Cal_sys/9(KeSMSw4SAcsMd26FwdBkwdTrgtPosCalib_TrgtPosArray_write) -> KeSMSw4SAcsMd26FwdBkwdTrgtPosCalib_TrgtPosArray/1
  SecRwLtStFwdBkwdTrgtPosSelc_1_Cal_sys/10(KeSMSw4sLegrstOpenLMdFwdBkwdTrgtPosCalib_TrgtPosArray_write) -> KeSMSw4sLegrstOpenLMdFwdBkwdTrgtPosCalib_TrgtPosArray/1
  SecRwLtStFwdBkwdTrgtPosSelc_1_Cal_sys/11(KeSMSw4SLyingLMDFwdBkwdTrgtPosCalib_TrgtPosArray_write) -> KeSMSw4SLyingLMDFwdBkwdTrgtPosCalib_TrgtPosArray/1
  SecRwLtStFwdBkwdTrgtPosSelc_1_Cal_sys/12(KeSMSw4SVIPLMDFwdBkwdTrgtPosCalib_TrgtPosArray_write) -> KeSMSw4SVIPLMDFwdBkwdTrgtPosCalib_TrgtPosArray/1
  SecRwLtStFwdBkwdTrgtPosSelc_1_Cal_sys/13(Md56R2LFwdBkwdTrgtPosCalib_TrgtPosArray_write) -> Md56R2LFwdBkwdTrgtPosCalib_TrgtPosArray/1
  SecRwLtStFwdBkwdTrgtPosSelc_1_Cal_sys/14(Md8R2LFwdBkwdTrgtPosCalib_TrgtPosArray_write) -> Md8R2LFwdBkwdTrgtPosCalib_TrgtPosArray/1
  SecRwLtStFwdBkwdTrgtPosSelc_1_Cal_sys/15(SecRwLtStFwdBkwdEnTrigBitMask_Val_write) -> SecRwLtStFwdBkwdEnTrigBitMask_Val/1
  SecRwLtStFwdBkwdTrgtPosSelc_1_Cal_sys/16(VIPLExitR2LFwdBkwdTrgtPosCalib_TrgtPosArray_write) -> VIPLExitR2LFwdBkwdTrgtPosCalib_TrgtPosArray/1
  SecRwLtStFwdBkwdTrgtPosSelc_1_Cal_sys/17(VIPLR2LFwdBkwdTrgtPosCalib_TrgtPosArray_write) -> VIPLR2LFwdBkwdTrgtPosCalib_TrgtPosArray/1
  SecRwLtStHdrstFwdBkwdTrgtPosSelc_1_Cal_sys/1(KeSMSw4SAcsMd21HdrstFwdBkwdTrgtPosCalib_TrgtPosArray_write) -> KeSMSw4SAcsMd21HdrstFwdBkwdTrgtPosCalib_TrgtPosArray/1
  SecRwLtStHdrstFwdBkwdTrgtPosSelc_1_Cal_sys/2(KeSMSw4SAcsMd22HdrstFwdBkwdTrgtPosCalib_TrgtPosArray_write) -> KeSMSw4SAcsMd22HdrstFwdBkwdTrgtPosCalib_TrgtPosArray/1
  SecRwLtStHdrstFwdBkwdTrgtPosSelc_1_Cal_sys/3(KeSMSw4SAcsMd25HdrstFwdBkwdTrgtPosCalib_TrgtPosArray_write) -> KeSMSw4SAcsMd25HdrstFwdBkwdTrgtPosCalib_TrgtPosArray/1
  SecRwLtStHdrstFwdBkwdTrgtPosSelc_1_Cal_sys/4(KeSMSw4SAcsMd26HdrstFwdBkwdTrgtPosCalib_TrgtPosArray_write) -> KeSMSw4SAcsMd26HdrstFwdBkwdTrgtPosCalib_TrgtPosArray/1
  SecRwLtStHdrstFwdBkwdTrgtPosSelc_1_Cal_sys/5(LyLR2LHdrstFwdBkwdTrgtPosCalib_TrgtPosArray_write) -> LyLR2LHdrstFwdBkwdTrgtPosCalib_TrgtPosArray/1
  SecRwLtStHdrstFwdBkwdTrgtPosSelc_1_Cal_sys/6(RecvLR2LHdrstFwdBkwdTrgtPosCalib_TrgtPosArray_write) -> RecvLR2LHdrstFwdBkwdTrgtPosCalib_TrgtPosArray/1
  SecRwLtStHdrstFwdBkwdTrgtPosSelc_1_Cal_sys/7(VIPLR2LHdrstFwdBkwdTrgtPosCalib_TrgtPosArray_write) -> VIPLR2LHdrstFwdBkwdTrgtPosCalib_TrgtPosArray/1
  SecRwLtStHdrstUpwdDnwdTrgtPosSelc_1_Cal_sys/1(KeSMSw4SAcsMd21HdrstUpwdDnwdTrgtPosCalib_TrgtPosArray_write) -> KeSMSw4SAcsMd21HdrstUpwdDnwdTrgtPosCalib_TrgtPosArray/1
  SecRwLtStHdrstUpwdDnwdTrgtPosSelc_1_Cal_sys/2(KeSMSw4SAcsMd22HdrstUpwdDnwdTrgtPosCalib_TrgtPosArray_write) -> KeSMSw4SAcsMd22HdrstUpwdDnwdTrgtPosCalib_TrgtPosArray/1
  SecRwLtStHdrstUpwdDnwdTrgtPosSelc_1_Cal_sys/3(KeSMSw4SAcsMd25HdrstUpwdDnwdTrgtPosCalib_TrgtPosArray_write) -> KeSMSw4SAcsMd25HdrstUpwdDnwdTrgtPosCalib_TrgtPosArray/1
  SecRwLtStHdrstUpwdDnwdTrgtPosSelc_1_Cal_sys/4(KeSMSw4SAcsMd26HdrstUpwdDnwdTrgtPosCalib_TrgtPosArray_write) -> KeSMSw4SAcsMd26HdrstUpwdDnwdTrgtPosCalib_TrgtPosArray/1
  SecRwLtStHdrstUpwdDnwdTrgtPosSelc_1_Cal_sys/5(LyLR2LHdrstUpwdDnwdTrgtPosCalib_TrgtPosArray_write) -> LyLR2LHdrstUpwdDnwdTrgtPosCalib_TrgtPosArray/1
  SecRwLtStHdrstUpwdDnwdTrgtPosSelc_1_Cal_sys/6(RecvLR2LHdrstUpwdDnwdTrgtPosCalib_TrgtPosArray_write) -> RecvLR2LHdrstUpwdDnwdTrgtPosCalib_TrgtPosArray/1
  SecRwLtStHdrstUpwdDnwdTrgtPosSelc_1_Cal_sys/7(VIPLR2LHdrstUpwdDnwdTrgtPosCalib_TrgtPosArray_write) -> VIPLR2LHdrstUpwdDnwdTrgtPosCalib_TrgtPosArray/1
  SecRwLtStLgrstInwdOtwdTrgtPosSelc_1_Cal_sys/1(KeSMSw4SAcsMd22LgrstInwdOtwdTrgtPosCalib_TrgtPosArray_write) -> KeSMSw4SAcsMd22LgrstInwdOtwdTrgtPosCalib_TrgtPosArray/1
  SecRwLtStLgrstInwdOtwdTrgtPosSelc_1_Cal_sys/2(KeSMSw4SAcsMd26LgrstInwdOtwdTrgtPosCalib_TrgtPosArray_write) -> KeSMSw4SAcsMd26LgrstInwdOtwdTrgtPosCalib_TrgtPosArray/1
  SecRwLtStLgrstInwdOtwdTrgtPosSelc_1_Cal_sys/3(KeSMSwEZEEntryLgrstInwdOtwdTrgtPosCalib_TrgtPosArray_write) -> KeSMSwEZEEntryLgrstInwdOtwdTrgtPosCalib_TrgtPosArray/1
  SecRwLtStLgrstInwdOtwdTrgtPosSelc_1_Cal_sys/4(LgrstCloseLR2LLgrstInwdOtwdTrgtPosCalib_TrgtPosArray_write) -> LgrstCloseLR2LLgrstInwdOtwdTrgtPosCalib_TrgtPosArray/1
  SecRwLtStLgrstInwdOtwdTrgtPosSelc_1_Cal_sys/5(LgrstOpen4sLR2LLgrstInwdOtwdTrgtPosCalib_TrgtPosArray_write) -> LgrstOpen4sLR2LLgrstInwdOtwdTrgtPosCalib_TrgtPosArray/1
  SecRwLtStLgrstInwdOtwdTrgtPosSelc_1_Cal_sys/6(LyLR2LLgrstInwdOtwdTrgtPosCalib_TrgtPosArray_write) -> LyLR2LLgrstInwdOtwdTrgtPosCalib_TrgtPosArray/1
  SecRwLtStLgrstInwdOtwdTrgtPosSelc_1_Cal_sys/7(Md56LgrstInwdOtwdTrgtPosCalib_TrgtPosArray_write) -> Md56LgrstInwdOtwdTrgtPosCalib_TrgtPosArray/1
  SecRwLtStLgrstInwdOtwdTrgtPosSelc_1_Cal_sys/8(Md8R2LLgrstInwdOtwdTrgtPosCalib_TrgtPosArray_write) -> Md8R2LLgrstInwdOtwdTrgtPosCalib_TrgtPosArray/1
  SecRwLtStLgrstInwdOtwdTrgtPosSelc_1_Cal_sys/9(RecvLR2LLgrstInwdOtwdTrgtPosCalib_TrgtPosArray_write) -> RecvLR2LLgrstInwdOtwdTrgtPosCalib_TrgtPosArray/1
  SecRwLtStLgrstInwdOtwdTrgtPosSelc_1_Cal_sys/10(SecRwLtStLgrstInwdOtwdEnTrigBitMask_Val_write) -> SecRwLtStLgrstInwdOtwdEnTrigBitMask_Val/1
  SecRwLtStLgrstInwdOtwdTrgtPosSelc_1_Cal_sys/11(VIP4sLR2LLgrstInwdOtwdTrgtPosCalib_TrgtPosArray_write) -> VIP4sLR2LLgrstInwdOtwdTrgtPosCalib_TrgtPosArray/1
  SecRwLtStLgrstInwdOtwdTrgtPosSelc_1_Cal_sys/12(VIPLExitR2LLgrstInwdOtwdTrgtPosCalib_TrgtPosArray_write) -> VIPLExitR2LLgrstInwdOtwdTrgtPosCalib_TrgtPosArray/1
  SecRwLtStLgrstInwdOtwdTrgtPosSelc_1_Cal_sys/13(VIPLR2LLgrstInwdOtwdTrgtPosCalib_TrgtPosArray_write) -> VIPLR2LLgrstInwdOtwdTrgtPosCalib_TrgtPosArray/1
  SecRwLtStLgrstUpwdDnwdTrgtPosSelc_1_Cal_sys/1(EZER2LLgrstUpwdDnwdTrgtPosCalib_TrgtPosArray_write) -> EZER2LLgrstUpwdDnwdTrgtPosCalib_TrgtPosArray/1
  SecRwLtStLgrstUpwdDnwdTrgtPosSelc_1_Cal_sys/2(EZQR2LLgrstUpwdDnwdTrgtPosCalib_TrgtPosArray_write) -> EZQR2LLgrstUpwdDnwdTrgtPosCalib_TrgtPosArray/1
  SecRwLtStLgrstUpwdDnwdTrgtPosSelc_1_Cal_sys/3(KeSMSw4SAcsMd22LgrstUpwdDnwdTrgtPosCalib_TrgtPosArray_write) -> KeSMSw4SAcsMd22LgrstUpwdDnwdTrgtPosCalib_TrgtPosArray/1
  SecRwLtStLgrstUpwdDnwdTrgtPosSelc_1_Cal_sys/4(KeSMSw4SAcsMd26LgrstUpwdDnwdTrgtPosCalib_TrgtPosArray_write) -> KeSMSw4SAcsMd26LgrstUpwdDnwdTrgtPosCalib_TrgtPosArray/1
  SecRwLtStLgrstUpwdDnwdTrgtPosSelc_1_Cal_sys/5(LgrstCloseLR2LLgrstUpwdDnwdTrgtPosCalib_TrgtPosArray_write) -> LgrstCloseLR2LLgrstUpwdDnwdTrgtPosCalib_TrgtPosArray/1
  SecRwLtStLgrstUpwdDnwdTrgtPosSelc_1_Cal_sys/6(LgrstOpenLR2LLgrstUpwdDnwdTrgtPosCalib_TrgtPosArray_write) -> LgrstOpenLR2LLgrstUpwdDnwdTrgtPosCalib_TrgtPosArray/1
  SecRwLtStLgrstUpwdDnwdTrgtPosSelc_1_Cal_sys/7(LyLR2LLgrstUpwdDnwdTrgtPosCalib_TrgtPosArray_write) -> LyLR2LLgrstUpwdDnwdTrgtPosCalib_TrgtPosArray/1
  SecRwLtStLgrstUpwdDnwdTrgtPosSelc_1_Cal_sys/8(Md56R2LLgrstUpwdDnwdTrgtPosCalib_TrgtPosArray_write) -> Md56R2LLgrstUpwdDnwdTrgtPosCalib_TrgtPosArray/1
  SecRwLtStLgrstUpwdDnwdTrgtPosSelc_1_Cal_sys/9(Md8R2LLgrstUpwdDnwdTrgtPosCalib_TrgtPosArray_write) -> Md8R2LLgrstUpwdDnwdTrgtPosCalib_TrgtPosArray/1
  SecRwLtStLgrstUpwdDnwdTrgtPosSelc_1_Cal_sys/10(RecvLR2LLgrstUpwdDnwdTrgtPosCalib_TrgtPosArray_write) -> RecvLR2LLgrstUpwdDnwdTrgtPosCalib_TrgtPosArray/1
  SecRwLtStLgrstUpwdDnwdTrgtPosSelc_1_Cal_sys/11(SecRwLtStLgrstUpwdDnwdEnTrigBitMask_Val_write) -> SecRwLtStLgrstUpwdDnwdEnTrigBitMask_Val/1
  SecRwLtStLgrstUpwdDnwdTrgtPosSelc_1_Cal_sys/12(VIPExitLR2LLgrstUpwdDnwdTrgtPosCalib_TrgtPosArray_write) -> VIPExitLR2LLgrstUpwdDnwdTrgtPosCalib_TrgtPosArray/1
  SecRwLtStLgrstUpwdDnwdTrgtPosSelc_1_Cal_sys/13(VIPLR2LLgrstUpwdDnwdTrgtPosCalib_TrgtPosArray_write) -> VIPLR2LLgrstUpwdDnwdTrgtPosCalib_TrgtPosArray/1
  SecRwLtStLtwdRtwdTrgtPosSelc_1_Cal_sys/1(EZER2LLtwdRtwdTrgtPosCalib_TrgtPosArray_write) -> EZER2LLtwdRtwdTrgtPosCalib_TrgtPosArray/1
  SecRwLtStLtwdRtwdTrgtPosSelc_1_Cal_sys/2(EZQR2LLtwdRtwdTrgtPosCalib_TrgtPosArray_write) -> EZQR2LLtwdRtwdTrgtPosCalib_TrgtPosArray/1
  SecRwLtStLtwdRtwdTrgtPosSelc_1_Cal_sys/3(FamlyLR2LLtwdRtwdTrgtPosCalib_TrgtPosArray_write) -> FamlyLR2LLtwdRtwdTrgtPosCalib_TrgtPosArray/1
  SecRwLtStLtwdRtwdTrgtPosSelc_1_Cal_sys/4(FamlyRR2LLtwdRtwdTrgtPosCalib_TrgtPosArray_write) -> FamlyRR2LLtwdRtwdTrgtPosCalib_TrgtPosArray/1
  SecRwLtStLtwdRtwdTrgtPosSelc_1_Cal_sys/5(INTMLR2LLtwdRtwdTrgtPosCalib_TrgtPosArray_write) -> INTMLR2LLtwdRtwdTrgtPosCalib_TrgtPosArray/1
  SecRwLtStLtwdRtwdTrgtPosSelc_1_Cal_sys/6(INTMRR2LLtwdRtwdTrgtPosCalib_TrgtPosArray_write) -> INTMRR2LLtwdRtwdTrgtPosCalib_TrgtPosArray/1
  SecRwLtStLtwdRtwdTrgtPosSelc_1_Cal_sys/7(VIPLR2LLtwdRtwdTrgtPosCalib_TrgtPosArray_write) -> VIPLR2LLtwdRtwdTrgtPosCalib_TrgtPosArray/1
  SecRwLtStZeroTrgtPosSelc_1_Cal_sys/1(ComfortMdR2LZeroTrgtPosCalib_TrgtPosArray_write) -> ComfortMdR2LZeroTrgtPosCalib_TrgtPosArray/1
  SecRwLtStZeroTrgtPosSelc_1_Cal_sys/2(EZEMdR2LZeroTrgtPosCalib_TrgtPosArray_write) -> EZEMdR2LZeroTrgtPosCalib_TrgtPosArray/1
  SecRwLtStZeroTrgtPosSelc_1_Cal_sys/3(Md56R2LZeroTrgtPosCalib_TrgtPosArray_write) -> Md56R2LZeroTrgtPosCalib_TrgtPosArray/1
  SecRwLtStZeroTrgtPosSelc_1_Cal_sys/4(Md8R2LZeroTrgtPosCalib_TrgtPosArray_write) -> Md8R2LZeroTrgtPosCalib_TrgtPosArray/1
  SecRwLtStZeroTrgtPosSelc_1_Cal_sys/5(SecRwLtStZeroEnTrigBitMask_Val_write) -> SecRwLtStZeroEnTrigBitMask_Val/1
  SecRwLtStZeroTrgtPosSelc_1_Cal_sys/6(SecRwLtStZeroTrgtPosCalibArray32_TrgtPosArray32_write) -> SecRwLtStZeroTrgtPosCalibArray32_TrgtPosArray32/1
  SecRwLtStZeroTrgtPosSelc_1_Cal_sys/7(VIPLExitMdR2LZeroTrgtPosCalib_TrgtPosArray_write) -> VIPLExitMdR2LZeroTrgtPosCalib_TrgtPosArray/1
  SecRwLtStZeroTrgtPosSelc_1_Cal_sys/8(VIPLMdR2LZeroTrgtPosCalib_TrgtPosArray_write) -> VIPLMdR2LZeroTrgtPosCalib_TrgtPosArray/1
  IfVeSMSuHeightIndexLt_Val/1 -> [IfVeSMSuHeightIndexLt_Val_Tag]
  [IfVeSMSuHeightIndexLt_Val_Tag] -> SecRwLtStHdrstFwdBkwdTrgtPosSelc_1_Cal_sys/1(IfVeSMSuHeightIndexLt_Val_read)
  [IfVeSMSuHeightIndexLt_Val_Tag] -> SecRwLtStHdrstUpwdDnwdTrgtPosSelc_1_Cal_sys/1(IfVeSMSuHeightIndexLt_Val_read)
  [IfVeSMSuHeightIndexLt_Val_Tag] -> SecRwLtStLgrstInwdOtwdTrgtPosSelc_1_Cal_sys/2(IfVeSMSuHeightIndexLt_Val_read)
  IfVeSMSbSecRwLtStCshnFrntUpwdDnwdMovConfig_Val/1 -> [IfVeSMSbSecRwLtStCshnFrntUpwdDnwdMovConfig_Val_Tag]
  [IfVeSMSbSecRwLtStCshnFrntUpwdDnwdMovConfig_Val_Tag] -> SecRwLtStBkReclnTrgtPosSelc_1_Cal_sys/1(IfVeSMSbSecRwLtStCshnFrntUpwdDnwdMovConfig_Val_read)
  [IfVeSMSbSecRwLtStCshnFrntUpwdDnwdMovConfig_Val_Tag] -> SecRwLtStFwdBkwdTrgtPosSelc_1_Cal_sys/1(IfVeSMSbSecRwLtStCshnFrntUpwdDnwdMovConfig_Val_read)
  [IfVeSMSbSecRwLtStCshnFrntUpwdDnwdMovConfig_Val_Tag] -> SecRwLtStLgrstInwdOtwdTrgtPosSelc_1_Cal_sys/1(IfVeSMSbSecRwLtStCshnFrntUpwdDnwdMovConfig_Val_read)
  [IfVeSMSbSecRwLtStCshnFrntUpwdDnwdMovConfig_Val_Tag] -> SecRwLtStLgrstUpwdDnwdTrgtPosSelc_1_Cal_sys/1(IfVeSMSbSecRwLtStCshnFrntUpwdDnwdMovConfig_Val_read)
  StNumFlg_Is7s/1 -> [StNumFlg_Is7s_Tag]
  [StNumFlg_Is7s_Tag] -> SecRwLtStArmScrnTrgtPosSelc_1_Cal_sys/4(StNumFlg_Is7s_read)
  [StNumFlg_Is7s_Tag] -> SecRwLtStBkReclnTrgtPosSelc_1_Cal_sys/9(StNumFlg_Is7s_read)
  [StNumFlg_Is7s_Tag] -> SecRwLtStFtrstTrgtPosSelc_1_Cal_sys/4(StNumFlg_Is7s_read)
  [StNumFlg_Is7s_Tag] -> SecRwLtStFwdBkwdTrgtPosSelc_1_Cal_sys/7(StNumFlg_Is7s_read)
  [StNumFlg_Is7s_Tag] -> SecRwLtStHdrstFwdBkwdTrgtPosSelc_1_Cal_sys/5(StNumFlg_Is7s_read)
  [StNumFlg_Is7s_Tag] -> SecRwLtStHdrstUpwdDnwdTrgtPosSelc_1_Cal_sys/5(StNumFlg_Is7s_read)
  [StNumFlg_Is7s_Tag] -> SecRwLtStLgrstInwdOtwdTrgtPosSelc_1_Cal_sys/6(StNumFlg_Is7s_read)
  [StNumFlg_Is7s_Tag] -> SecRwLtStLgrstUpwdDnwdTrgtPosSelc_1_Cal_sys/5(StNumFlg_Is7s_read)
  [StNumFlg_Is7s_Tag] -> SecRwLtStLtwdRtwdTrgtPosSelc_1_Cal_sys/4(StNumFlg_Is7s_read)
  [StNumFlg_Is7s_Tag] -> SecRwLtStZeroTrgtPosSelc_1_Cal_sys/4(StNumFlg_Is7s_read)
  StNumFlg_Is6s7s/1 -> [StNumFlg_Is6s7s_Tag]
  [StNumFlg_Is6s7s_Tag] -> SecRwLtStArmScrnTrgtPosSelc_1_Cal_sys/3(StNumFlg_Is6s7s_read)
  [StNumFlg_Is6s7s_Tag] -> SecRwLtStBkReclnTrgtPosSelc_1_Cal_sys/8(StNumFlg_Is6s7s_read)
  [StNumFlg_Is6s7s_Tag] -> SecRwLtStFtrstTrgtPosSelc_1_Cal_sys/3(StNumFlg_Is6s7s_read)
  [StNumFlg_Is6s7s_Tag] -> SecRwLtStFwdBkwdTrgtPosSelc_1_Cal_sys/6(StNumFlg_Is6s7s_read)
  [StNumFlg_Is6s7s_Tag] -> SecRwLtStHdrstFwdBkwdTrgtPosSelc_1_Cal_sys/4(StNumFlg_Is6s7s_read)
  [StNumFlg_Is6s7s_Tag] -> SecRwLtStHdrstUpwdDnwdTrgtPosSelc_1_Cal_sys/4(StNumFlg_Is6s7s_read)
  [StNumFlg_Is6s7s_Tag] -> SecRwLtStLgrstInwdOtwdTrgtPosSelc_1_Cal_sys/5(StNumFlg_Is6s7s_read)
  [StNumFlg_Is6s7s_Tag] -> SecRwLtStLgrstUpwdDnwdTrgtPosSelc_1_Cal_sys/4(StNumFlg_Is6s7s_read)
  [StNumFlg_Is6s7s_Tag] -> SecRwLtStLtwdRtwdTrgtPosSelc_1_Cal_sys/3(StNumFlg_Is6s7s_read)
  [StNumFlg_Is6s7s_Tag] -> SecRwLtStZeroTrgtPosSelc_1_Cal_sys/3(StNumFlg_Is6s7s_read)
  StNumFlg_Is6s/1 -> [StNumFlg_Is6s_Tag]
  [StNumFlg_Is6s_Tag] -> SecRwLtStArmScrnTrgtPosSelc_1_Cal_sys/2(StNumFlg_Is6s_read)
  [StNumFlg_Is6s_Tag] -> SecRwLtStBkReclnTrgtPosSelc_1_Cal_sys/7(StNumFlg_Is6s_read)
  [StNumFlg_Is6s_Tag] -> SecRwLtStFtrstTrgtPosSelc_1_Cal_sys/2(StNumFlg_Is6s_read)
  [StNumFlg_Is6s_Tag] -> SecRwLtStFwdBkwdTrgtPosSelc_1_Cal_sys/5(StNumFlg_Is6s_read)
  [StNumFlg_Is6s_Tag] -> SecRwLtStHdrstFwdBkwdTrgtPosSelc_1_Cal_sys/3(StNumFlg_Is6s_read)
  [StNumFlg_Is6s_Tag] -> SecRwLtStHdrstUpwdDnwdTrgtPosSelc_1_Cal_sys/3(StNumFlg_Is6s_read)
  [StNumFlg_Is6s_Tag] -> SecRwLtStLgrstInwdOtwdTrgtPosSelc_1_Cal_sys/4(StNumFlg_Is6s_read)
  [StNumFlg_Is6s_Tag] -> SecRwLtStLgrstUpwdDnwdTrgtPosSelc_1_Cal_sys/3(StNumFlg_Is6s_read)
  [StNumFlg_Is6s_Tag] -> SecRwLtStLtwdRtwdTrgtPosSelc_1_Cal_sys/2(StNumFlg_Is6s_read)
  [StNumFlg_Is6s_Tag] -> SecRwLtStZeroTrgtPosSelc_1_Cal_sys/2(StNumFlg_Is6s_read)
  StNumFlg_Is4s/1 -> [StNumFlg_Is4s_Tag]
  [StNumFlg_Is4s_Tag] -> SecRwLtStArmScrnTrgtPosSelc_1_Cal_sys/1(StNumFlg_Is4s_read)
  [StNumFlg_Is4s_Tag] -> SecRwLtStBkReclnTrgtPosSelc_1_Cal_sys/6(StNumFlg_Is4s_read)
  [StNumFlg_Is4s_Tag] -> SecRwLtStFtrstTrgtPosSelc_1_Cal_sys/1(StNumFlg_Is4s_read)
  [StNumFlg_Is4s_Tag] -> SecRwLtStFwdBkwdTrgtPosSelc_1_Cal_sys/4(StNumFlg_Is4s_read)
  [StNumFlg_Is4s_Tag] -> SecRwLtStHdrstFwdBkwdTrgtPosSelc_1_Cal_sys/2(StNumFlg_Is4s_read)
  [StNumFlg_Is4s_Tag] -> SecRwLtStHdrstUpwdDnwdTrgtPosSelc_1_Cal_sys/2(StNumFlg_Is4s_read)
  [StNumFlg_Is4s_Tag] -> SecRwLtStLgrstInwdOtwdTrgtPosSelc_1_Cal_sys/3(StNumFlg_Is4s_read)
  [StNumFlg_Is4s_Tag] -> SecRwLtStLgrstUpwdDnwdTrgtPosSelc_1_Cal_sys/2(StNumFlg_Is4s_read)
  [StNumFlg_Is4s_Tag] -> SecRwLtStLtwdRtwdTrgtPosSelc_1_Cal_sys/1(StNumFlg_Is4s_read)
  [StNumFlg_Is4s_Tag] -> SecRwLtStZeroTrgtPosSelc_1_Cal_sys/1(StNumFlg_Is4s_read)
  Md61SecRwRtStCushFrntTrgtPosCalib_TrgtPosArray/1 -> SecRwLtStZeroTrgtPosSelc_1_Cal_sys/5(Md61SecRwRtStCushFrntTrgtPosCalib_TrgtPosArray_read)
  Md62SecRwLtStCushFrntTrgtPosCalib_TrgtPosArray/1 -> SecRwLtStZeroTrgtPosSelc_1_Cal_sys/6(Md62SecRwLtStCushFrntTrgtPosCalib_TrgtPosArray_read)
  Md27Target1_Val/1 -> SecRwLtStBkReclnTrgtPosSelc_1_Cal_sys/11(Md27Target1_Val_read)
  Md27Target2_Val/1 -> SecRwLtStBkReclnTrgtPosSelc_1_Cal_sys/12(Md27Target2_Val_read)
  SecRwLtStBkReclnTrgtPosSelc_1_Cal_sys/17(Md27SecRwLtStBkReclnTrgtPosCalib_TrgtPosArray_write) -> Md27SecRwLtStBkReclnTrgtPosCalib_TrgtPosArray/1
